simulink model "likestromsmotor"  (R2017b)
settings: Solver=VariableStepAuto  StartTime=0.0  StopTime=simtime  RelTol=1e-3
values from neighbouring files (symbols this model uses):
  d = [T1 1 0]    [oppg2.m]
  n = [K]    [oppg2.m]
  y0 = 1    [oppg2.m]
settings Model: Creator=bendi  LastModifiedBy=bruker

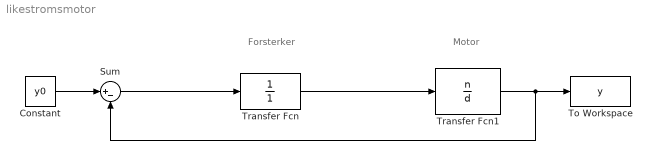
== system likestromsmotor ==
  note: Motor
  note: Forsterker
  Constant : Constant  Value=y0
  Sum : Sum  Inputs=|+-
  To Workspace : ToWorkspace  VariableName=y  SaveFormat=Timeseries  SampleTime=-1
  Transfer Fcn : TransferFcn  Denominator=[1]
  Transfer Fcn1 : TransferFcn  Numerator=n  Denominator=d
  wires:
  Sum/1 -> Transfer Fcn/1
  Constant/1 -> Sum/1
  Transfer Fcn1/1 -> Sum/2, To Workspace/1
  Transfer Fcn/1 -> Transfer Fcn1/1
